simulink model "VehV_DD"  (R2016b)
settings: configuration reference "CodeGenConfigSet" (kept outside this file)
values from neighbouring files (symbols this model uses):
  VehV_bSwtPrs_C = Calibration.Parameter    [init_VehV_DD.m]    (also in init_VehV_DD_SIL.m = Simulink.Parameter)
  VehV_ImpPerDist_C = Calibration.Parameter    [init_VehV_DD.m]    (also in init_VehV_DD_SIL.m = Simulink.Parameter)
  VehV_numImpCrdSh_C = Calibration.Parameter    [init_VehV_DD.m]    (also in init_VehV_DD_SIL.m = Simulink.Parameter)
settings Model: Creator=lenovo  LastModifiedBy=lenovo
settings ConfigSetRef: SourceLocation=Base Workspace

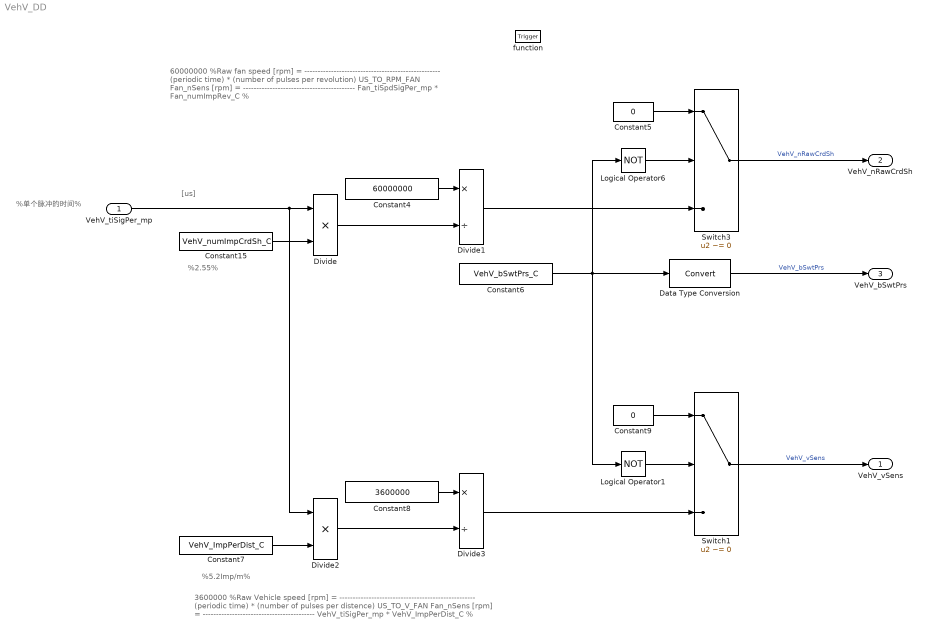
== system VehV_DD ==
  note: 3600000
      | %Raw Vehicle speed [rpm] = ---------------------------------------------------
      | (periodic time) * (number of pulses per distence)
      |
      | US_TO_V_FAN
      | Fan_nSens [rpm] = ------------------------------------------
      | VehV_tiSigPer_mp * VehV_ImpPerDist_C %
  note: 60000000
      | %Raw fan speed [rpm] = ---------------------------------------------------
      | (periodic time) * (number of pulses per revolution)
      |
      | US_TO_RPM_FAN
      | Fan_nSens [rpm] = ------------------------------------------
      | Fan_tiSpdSigPer_mp * Fan_numImpRev_C %
  note: [us]
  note: %2.55%
  note: %5.2Imp/m%
  note: %单个脉冲的时间%
  VehV_tiSigPer_mp : Inport  Tag=us  Description=signal period duration  OutMin=0  OutMax=6553  OutDataTypeStr=Period_us
  function : TriggerPort  TriggerType=function-call  VariantControl=Variant
  Constant15 : Constant  Value=VehV_numImpCrdSh_C
  Constant4 : Constant  Value=60000000  OutDataTypeStr=uint32
  Constant5 : Constant  Value=0  OutDataTypeStr=Inherit: Inherit via back propagation
  Constant6 : Constant  Value=VehV_bSwtPrs_C
  Constant7 : Constant  Value=VehV_ImpPerDist_C
  Constant8 : Constant  Value=3600000  OutDataTypeStr=uint32
  Constant9 : Constant  Value=0  OutDataTypeStr=Inherit: Inherit via back propagation
  Data Type Conversion : DataTypeConversion
  Divide : Product  Inputs=**  SaturateOnIntegerOverflow=on
  Divide1 : Product  Inputs=*/  OutDataTypeStr=Inherit: Inherit via back propagation  SaturateOnIntegerOverflow=on
  Divide2 : Product  Inputs=**  SaturateOnIntegerOverflow=on
  Divide3 : Product  Inputs=*/  OutDataTypeStr=Inherit: Inherit via back propagation  SaturateOnIntegerOverflow=on
  Logical Operator1 : Logic  Operator=NOT  OutDataTypeStr=boolean
  Logical Operator6 : Logic  Operator=NOT  OutDataTypeStr=boolean
  Switch1 : Switch  Criteria=u2 ~= 0  OutDataTypeStr=Inherit: Inherit via back propagation  SaturateOnIntegerOverflow=on  InputSameDT=on
  Switch3 : Switch  Criteria=u2 ~= 0  OutDataTypeStr=Inherit: Inherit via back propagation  SaturateOnIntegerOverflow=on  InputSameDT=on
  VehV_vSens : Outport  Tag=km/h  Description=Sensed vehicle speed  OutMin=0  OutMax=250  OutDataTypeStr=VehSpeed_km_h
  VehV_nRawCrdSh : Outport  Tag=rpm  Description=Raw Cardan shaft speed  Port=2  OutMin=0  OutMax=6000  OutDataTypeStr=EngSpeed_rpm
  VehV_bSwtPrs : Outport  Description=sensor switch  Port=3  OutMin=0  OutMax=1  OutDataTypeStr=boolean
  wires:
  Switch1/1 -> VehV_vSens/1  "VehV_vSens"
  Logical Operator1/1 -> Switch1/2
  Constant6/1 -> Data Type Conversion/1, Logical Operator6/1, Logical Operator1/1
  Divide3/1 -> Switch1/3
  Constant9/1 -> Switch1/1
  Divide2/1 -> Divide3/2
  Constant8/1 -> Divide3/1
  Constant7/1 -> Divide2/2
  Logical Operator6/1 -> Switch3/2
  Divide1/1 -> Switch3/3
  Divide/1 -> Divide1/2
  Constant4/1 -> Divide1/1
  VehV_tiSigPer_mp/1 -> Divide/1, Divide2/1
  Constant5/1 -> Switch3/1
  Constant15/1 -> Divide/2
  Switch3/1 -> VehV_nRawCrdSh/1  "VehV_nRawCrdSh"
  Data Type Conversion/1 -> VehV_bSwtPrs/1  "VehV_bSwtPrs"
